simulink model "IBVS"  (R2020a)
settings: Solver=VariableStepAuto  StartTime=0.0  StopTime=10.0  RelTol=1e-3
values from neighbouring files (symbols this model uses):
  f = 0.015    [camera.m]    (also in init.m = 0.05)
  O = [0; 0; 0]    [camera.m]    (also in init.m; sistemi_di_riferimento.m = [0;0;0])
  p = [4.6; 0.25; 1.8]    [camera.m]    (also in init.m = [1.0; 0.15; 0.8])
settings Model: Creator=Acer  LastModifiedBy=Acer

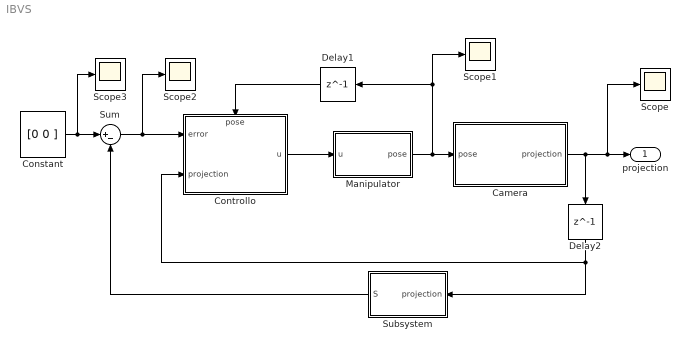
== system IBVS ==
  Camera : Subsystem
  Constant : Constant  Value=[0 0 ]  SampleTime=1/200
  Controllo : Subsystem
      settings: PortSchema="{\"entries\":[{\"content\":{\"sides\":[{\"content\":{\"connectorIds\":[\"In1\",\"In2\"]},\"type\":\"ConnectorPlacement.EquallySpacedRectSide\",\"uuid\":\"84d820fc-7a87-4e3d-8c01-2ff03d79ee5e\"},{\"content\":{\"connectorIds\":[\"Out1\"],\"side\":\"RIGHT\"},\"type\":\"ConnectorPlacement.EquallySpacedRectSide\",\"uuid\":\"415320e6-3d50-448c-a9e4-72393bfc9545\"},{\"content\":{\"connectorIds\":[\"In3\"],\"side\":\"TOP\"},\"type\":\"ConnectorPlacement.EquallySpacedRectSide\",\"uuid\":\"a0afcb71-1d8e-4c1f-85b7-12dcc8878713\"}]},\"type\":\"ConnectorPlacement.EquallySpacedConnector\",\"uuid\":\"9a74b34d-4794-49ec-9f78-f6fc4c4f61de\"}],\"packageUris\":[\"http://schema.mathworks.com/mf0/Connector/19700101\"],\"version\":\"1.0\"}"
  Delay1 : Delay  DelayLength=1
  Delay2 : Delay  DelayLength=1
  Manipulator : Subsystem
  Scope{,1..3} (4 alike) : Scope
  Subsystem : Subsystem
  Sum : Sum  Inputs=|+-
  projection : Outport
  wires:
  Camera/1(projection) -> Scope/1, projection/1, Delay2/1
  Controllo/1(u) -> Manipulator/1(u)
  Manipulator/1(pose) -> Scope1/1, Delay1/1, Camera/1(pose)
  Constant/1 -> Scope3/1, Sum/1
  Sum/1 -> Scope2/1, Controllo/1(error)
  Delay1/1 -> Controllo/3(pose)
  Subsystem/1(S) -> Sum/2
  Delay2/1 -> Subsystem/1(projection), Controllo/2(projection)

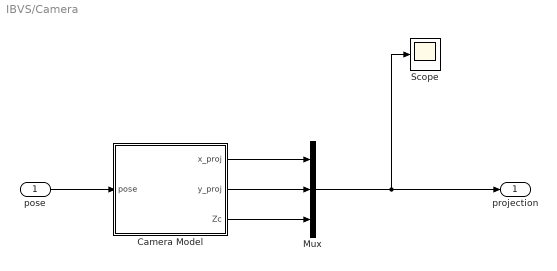
== system IBVS/Camera ==
  pose : Inport
  Camera Model : MATLAB Function  TreatAsAtomicUnit=on  SystemSampleTime=1/200
  Mux : Mux  Inputs=3
  Scope : Scope
  projection : Outport
  wires:
  Mux/1 -> projection/1, Scope/1
  Camera Model/1(x_proj) -> Mux/1
  pose/1 -> Camera Model/1(pose)
  Camera Model/2(y_proj) -> Mux/2
  Camera Model/3(Zc) -> Mux/3

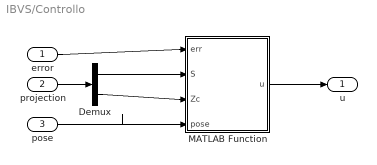
== system IBVS/Controllo ==
  error : Inport
  projection : Inport  Port=2
  pose : Inport  Port=3
  Demux : Demux  Outputs=[2, 1]
  MATLAB Function : MATLAB Function  TreatAsAtomicUnit=on  SystemSampleTime=1/200
  u : Outport
  wires:
  MATLAB Function/1(u) -> u/1
  projection/1 -> Demux/1
  Demux/2 -> MATLAB Function/3(Zc)
  Demux/1 -> MATLAB Function/2(S)
  error/1 -> MATLAB Function/1(err)
  pose/1 -> MATLAB Function/4(pose)

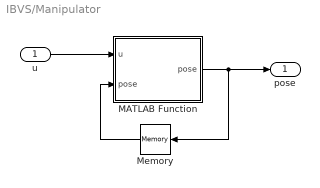
== system IBVS/Manipulator ==
  u : Inport
  MATLAB Function : MATLAB Function  TreatAsAtomicUnit=on  SystemSampleTime=1/200
  Memory : Memory  InitialCondition=zeros(6,1)
  pose : Outport
  wires:
  MATLAB Function/1(pose) -> Memory/1, pose/1
  u/1 -> MATLAB Function/1(u)
  Memory/1 -> MATLAB Function/2("pose ")

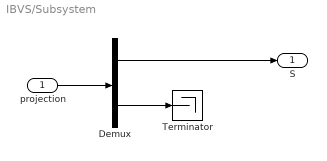
== system IBVS/Subsystem ==
  projection : Inport
  Demux : Demux  Outputs=[2, 1]
  Terminator : Terminator
  S : Outport
  wires:
  projection/1 -> Demux/1
  Demux/1 -> S/1
  Demux/2 -> Terminator/1

== matlab function IBVS/Controllo/MATLAB Function ==
  data: err input; S input; u output; Zc input; pose input; Kp parameter
function u = fcn(err, S, Zc, pose, Kp)

x = S(1);         % x projection in the image plane
y = S(2);         % y projection
ang = pose(4:6);  % camera's orientation 

Ls = [ -1/Zc 0 x/Zc x*y -(1+x^2) y;   % Interaction matrix
        0 -1/Zc y/Zc 1+y^2 -x*y -x];
Rx = [1   0       0   ;
      0 cos(ang(1)) -sin(ang(1));
      0 sin(ang(1)) cos(ang(1))];

Ry = [cos(ang(2)) 0 sin(ang(2)) ;
       0     1   0    ;
     -sin(ang(2)) 0 cos(ang(2))];
 
Rz = [cos(ang(3)) -sin(ang(3)) 0;
      sin(ang(3))  cos(ang(3)) 0;
       0      0     1];


Rc = Rx*Ry*Rz;
J = eye(6);
Jl = Ls*[Rc' zeros(3); zeros(3) Rc']*J;  
         
u = Jl'*Kp*err;

== matlab function IBVS/Camera/Camera Model ==
  data: x_proj output; y_proj output; Zc output; f parameter; p parameter; O parameter; pose input
function [x_proj, y_proj, Zc] = proj(f, p, O, pose)

d = pose(1:3) - O;    % camera's position in world frame
ang = pose(4:6);      % camera's orientation 
Twc = [rot(ang(1),ang(2),ang(3))   d;
                zeros(1,3)         1];

p_cam = Twc^-1 * [p;1];   % point's position in camera frame

P = diag([f,f,1]) * [eye(3), zeros(3,1)]; % camera projection matrix

p_tilde = P*p_cam;       
x_proj = -p_tilde(1)/p(3);
y_proj = p_tilde(2)/p(3);
Zc = p(3) - pose(3);

end

== matlab function IBVS/Manipulator/MATLAB Function ==
  data: u input; pose output; pose input; init_pose parameter
function pose = fcn(u, pose, init_pose)

if pose == zeros(6,1)    % initialization
pose = init_pose;
end

delta_t = 1/200;
pose = pose + u*delta_t;

end
